simulink model "UKF"  (R2020b)
settings: Solver=VariableStepAuto  StartTime=0.0  StopTime=100  RelTol=1e-3
values from neighbouring files (symbols this model uses):
  A = [0 1 0 0; 0 0 0 0; 0 0 0 omega; 0 0 -omega 0]    [one_sine_wave.m]    (also in two_sine_wave.m = [0 1 0 0 0 0)
  acc = 0    [one_sine_wave.m]    (also in two_sine_wave.m)
  H = 100    [one_sine_wave.m]    (also in two_sine_wave.m)
libraries: sharedTrackingLibrary x3, simulink x2
settings Model: Creator=Bruger  LastModifiedBy=Bruger

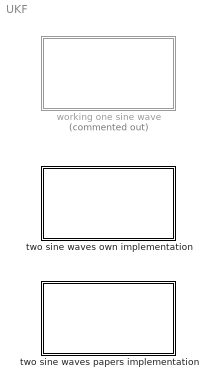
== system UKF ==
  two sine waves own implementation : Subsystem
  two sine waves papers implementation : Subsystem
  working one sine wave : Subsystem  Commented=on

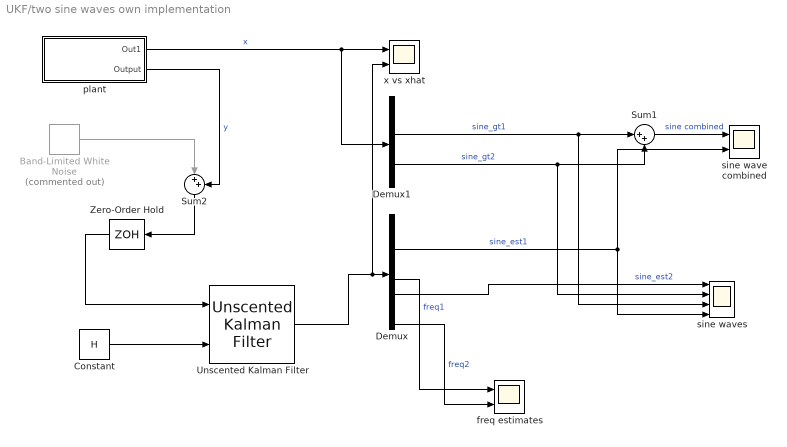
== system UKF/two sine waves own implementation ==
  Band-Limited White Noise : simulink/Sources/Band-Limited White Noise  Commented=on  Cov=[0.1]  Ts=0.05  seed=[23341]
  Constant : Constant  Value=H
  Demux : Demux  Outputs=8
  Demux1 : Demux  Outputs=6
  Sum1 : Sum  Inputs=|++
  Sum2 : Sum  Inputs=|++
  Unscented Kalman Filter : sharedTrackingLibrary/Unscented Kalman Filter  StateTransitionFcn=st_two_sine_own  HasAdditiveProcessNoise=Additive  ProcessNoise=0.1  HasTimeVaryingProcessNoise=off  HasStateTransitionFcnExtraArgument=0  InitialState=[100 0 0 20 0.5 0 40 1]  InitialStateCovariance=0.1  Alpha=1e-3  Beta=2  Kappa=0  MeasurementFcn1=meas_two_sine  HasMeasurementEnablePort1=off  HasAdditiveMeasurementNoise1=Additive  MeasurementNoise1=0.1  HasTimeVaryingMeasurementNoise1=off  HasMeasurementFcnExtraArgument1=0  MeasurementFcn2=measure_alt  HasMeasurementEnablePort2=off  HasAdditiveMeasurementNoise2=Additive  MeasurementNoise2=0.1  HasTimeVaryingMeasurementNoise2=off  HasMeasurementFcnExtraArgument2=0  MeasurementFcn3=myMeasurementFcn  HasMeasurementEnablePort3=off  HasAdditiveMeasurementNoise3=Additive  MeasurementNoise3=1  HasTimeVaryingMeasurementNoise3=off  HasMeasurementFcnExtraArgument3=0  MeasurementFcn4=myMeasurementFcn  HasMeasurementEnablePort4=off  HasAdditiveMeasurementNoise4=Additive  MeasurementNoise4=1  HasTimeVaryingMeasurementNoise4=off  HasMeasurementFcnExtraArgument4=0  MeasurementFcn5=myMeasurementFcn  HasMeasurementEnablePort5=off  HasAdditiveMeasurementNoise5=Additive  MeasurementNoise5=1  HasTimeVaryingMeasurementNoise5=off  HasMeasurementFcnExtraArgument5=0  EnableMultirate=off  StateTransitionFcnSampleTime=1  MeasurementFcn1SampleTime=1  MeasurementFcn2SampleTime=1  MeasurementFcn3SampleTime=1  MeasurementFcn4SampleTime=1  MeasurementFcn5SampleTime=1  UseCurrentEstimator=on  OutputStateCovariance=off  DataType=double  SampleTime=0.02  NumberOfMeasurements=2
      settings: SourceProductBaseCode=CT,DR,TF,ID,LP,NV,AR,RO,RR,UV,VE
  Zero-Order Hold : ZeroOrderHold  SampleTime=0.02
  freq estimates : Scope  NumInputPorts=2
  plant : Subsystem
  sine wave combined : Scope  NumInputPorts=2
  sine waves : Scope  NumInputPorts=4
  x vs xhat : Scope  NumInputPorts=2
  wires:
  Zero-Order Hold/1 -> Unscented Kalman Filter/1
  Unscented Kalman Filter/1 -> x vs xhat/2, Demux/1
  plant/1(Out1) -> x vs xhat/1, Demux1/1  "x"
  Constant/1 -> Unscented Kalman Filter/2
  Demux/6 -> sine waves/1  "sine_est2"
  Demux1/5 -> Sum1/2, sine waves/2  "sine_gt2"
  Demux/3 -> sine waves/4, sine wave combined/2  "sine_est1"
  Demux1/3 -> Sum1/1, sine waves/3  "sine_gt1"
  Demux/8 -> freq estimates/2  "freq2"
  Sum1/1 -> sine wave combined/1  "sine combined"
  Band-Limited White Noise/1 -> Sum2/1
  plant/2(Output) -> Sum2/2  "y"
  Sum2/1 -> Zero-Order Hold/1
  Demux/5 -> freq estimates/1  "freq1"

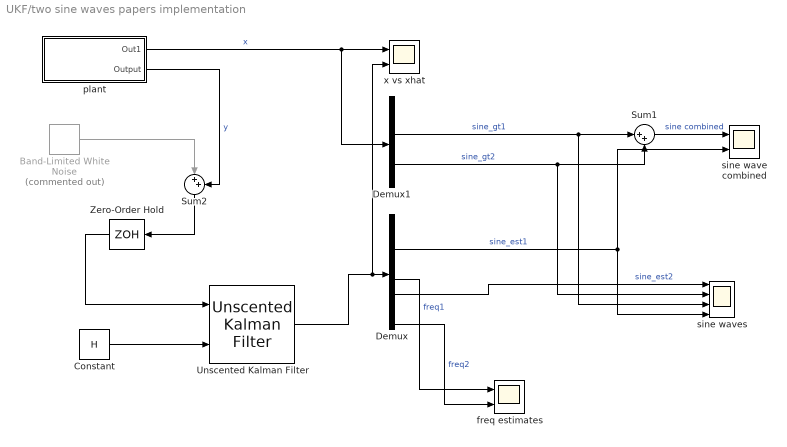
== system UKF/two sine waves papers implementation ==
  Band-Limited White Noise : simulink/Sources/Band-Limited White Noise  Commented=on  Cov=[0.1]  Ts=0.05  seed=[23341]
  Constant : Constant  Value=H
  Demux : Demux  Outputs=8
  Demux1 : Demux  Outputs=6
  Sum1 : Sum  Inputs=|++
  Sum2 : Sum  Inputs=|++
  Unscented Kalman Filter : sharedTrackingLibrary/Unscented Kalman Filter  StateTransitionFcn=st_two_sine_paper  HasAdditiveProcessNoise=Additive  ProcessNoise=0.1  HasTimeVaryingProcessNoise=off  HasStateTransitionFcnExtraArgument=0  InitialState=[100 0 0 20 0.5 0 40 1]  InitialStateCovariance=0.1  Alpha=1e-3  Beta=2  Kappa=0  MeasurementFcn1=meas_two_sine  HasMeasurementEnablePort1=off  HasAdditiveMeasurementNoise1=Additive  MeasurementNoise1=0.1  HasTimeVaryingMeasurementNoise1=off  HasMeasurementFcnExtraArgument1=0  MeasurementFcn2=measure_alt  HasMeasurementEnablePort2=off  HasAdditiveMeasurementNoise2=Additive  MeasurementNoise2=0.1  HasTimeVaryingMeasurementNoise2=off  HasMeasurementFcnExtraArgument2=0  MeasurementFcn3=myMeasurementFcn  HasMeasurementEnablePort3=off  HasAdditiveMeasurementNoise3=Additive  MeasurementNoise3=1  HasTimeVaryingMeasurementNoise3=off  HasMeasurementFcnExtraArgument3=0  MeasurementFcn4=myMeasurementFcn  HasMeasurementEnablePort4=off  HasAdditiveMeasurementNoise4=Additive  MeasurementNoise4=1  HasTimeVaryingMeasurementNoise4=off  HasMeasurementFcnExtraArgument4=0  MeasurementFcn5=myMeasurementFcn  HasMeasurementEnablePort5=off  HasAdditiveMeasurementNoise5=Additive  MeasurementNoise5=1  HasTimeVaryingMeasurementNoise5=off  HasMeasurementFcnExtraArgument5=0  EnableMultirate=off  StateTransitionFcnSampleTime=1  MeasurementFcn1SampleTime=1  MeasurementFcn2SampleTime=1  MeasurementFcn3SampleTime=1  MeasurementFcn4SampleTime=1  MeasurementFcn5SampleTime=1  UseCurrentEstimator=on  OutputStateCovariance=off  DataType=double  SampleTime=0.02  NumberOfMeasurements=2
      settings: SourceProductBaseCode=CT,DR,TF,ID,LP,NV,AR,RO,RR,UV,VE
  Zero-Order Hold : ZeroOrderHold  SampleTime=0.02
  freq estimates : Scope  NumInputPorts=2
  plant : Subsystem
  sine wave combined : Scope  NumInputPorts=2
  sine waves : Scope  NumInputPorts=4
  x vs xhat : Scope  NumInputPorts=2
  wires:
  Zero-Order Hold/1 -> Unscented Kalman Filter/1
  Unscented Kalman Filter/1 -> x vs xhat/2, Demux/1
  plant/1(Out1) -> x vs xhat/1, Demux1/1  "x"
  Constant/1 -> Unscented Kalman Filter/2
  Demux/6 -> sine waves/1  "sine_est2"
  Demux1/5 -> Sum1/2, sine waves/2  "sine_gt2"
  Demux/3 -> sine waves/4, sine wave combined/2  "sine_est1"
  Demux1/3 -> Sum1/1, sine waves/3  "sine_gt1"
  Demux/8 -> freq estimates/2  "freq2"
  Sum1/1 -> sine wave combined/1  "sine combined"
  Band-Limited White Noise/1 -> Sum2/1
  plant/2(Output) -> Sum2/2  "y"
  Sum2/1 -> Zero-Order Hold/1
  Demux/5 -> freq estimates/1  "freq1"

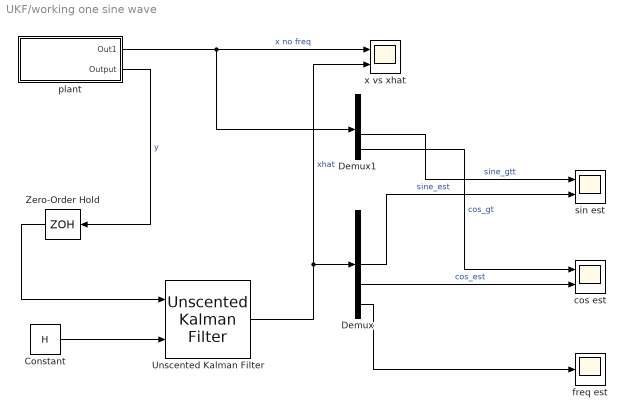
== system UKF/working one sine wave ==
  Constant : Constant  Value=H
  Demux : Demux  Outputs=5
  Demux1 : Demux
  Unscented Kalman Filter : sharedTrackingLibrary/Unscented Kalman Filter  StateTransitionFcn=st_one_sine  HasAdditiveProcessNoise=Additive  ProcessNoise=0.1  HasTimeVaryingProcessNoise=off  HasStateTransitionFcnExtraArgument=0  InitialState=[100 0 0 10 1]  InitialStateCovariance=0.1  Alpha=1e-3  Beta=2  Kappa=0  MeasurementFcn1=meas_one_sine  HasMeasurementEnablePort1=off  HasAdditiveMeasurementNoise1=Additive  MeasurementNoise1=0.1  HasTimeVaryingMeasurementNoise1=off  HasMeasurementFcnExtraArgument1=0  MeasurementFcn2=measure_alt  HasMeasurementEnablePort2=off  HasAdditiveMeasurementNoise2=Additive  MeasurementNoise2=0.1  HasTimeVaryingMeasurementNoise2=off  HasMeasurementFcnExtraArgument2=0  MeasurementFcn3=myMeasurementFcn  HasMeasurementEnablePort3=off  HasAdditiveMeasurementNoise3=Additive  MeasurementNoise3=1  HasTimeVaryingMeasurementNoise3=off  HasMeasurementFcnExtraArgument3=0  MeasurementFcn4=myMeasurementFcn  HasMeasurementEnablePort4=off  HasAdditiveMeasurementNoise4=Additive  MeasurementNoise4=1  HasTimeVaryingMeasurementNoise4=off  HasMeasurementFcnExtraArgument4=0  MeasurementFcn5=myMeasurementFcn  HasMeasurementEnablePort5=off  HasAdditiveMeasurementNoise5=Additive  MeasurementNoise5=1  HasTimeVaryingMeasurementNoise5=off  HasMeasurementFcnExtraArgument5=0  EnableMultirate=off  StateTransitionFcnSampleTime=1  MeasurementFcn1SampleTime=1  MeasurementFcn2SampleTime=1  MeasurementFcn3SampleTime=1  MeasurementFcn4SampleTime=1  MeasurementFcn5SampleTime=1  UseCurrentEstimator=on  OutputStateCovariance=off  DataType=double  SampleTime=0.1  NumberOfMeasurements=2
      settings: SourceProductBaseCode=CT,DR,TF,ID,LP,NV,AR,RO,RR,UV,VE
  Zero-Order Hold : ZeroOrderHold  SampleTime=0.1
  cos est : Scope  NumInputPorts=2
  freq est : Scope
  plant : Subsystem
  sin est : Scope  NumInputPorts=2
  x vs xhat : Scope  NumInputPorts=2
  wires:
  Zero-Order Hold/1 -> Unscented Kalman Filter/1
  plant/2(Output) -> Zero-Order Hold/1  "y"
  plant/1(Out1) -> x vs xhat/1, Demux1/1  "x no freq"
  Constant/1 -> Unscented Kalman Filter/2
  Unscented Kalman Filter/1 -> x vs xhat/2, Demux/1  "xhat"
  Demux1/4 -> cos est/1  "cos_gt"
  Demux/4 -> cos est/2  "cos_est"
  Demux1/3 -> sin est/1  "sine_gtt"
  Demux/3 -> sin est/2  "sine_est"
  Demux/5 -> freq est/1

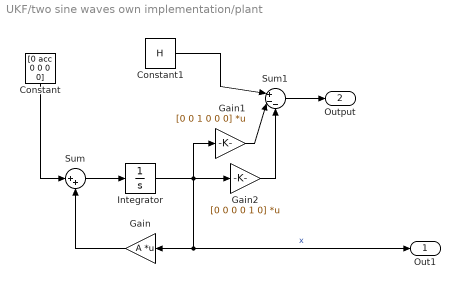
== system UKF/two sine waves own implementation/plant ==
  Constant : Constant  Value=[0 acc 0 0 0 0]
  Constant1 : Constant  Value=H
  Gain : Gain  Gain=A  Multiplication=Matrix(K*u) (u vector)
  Gain1 : Gain  Gain=[0 0 1 0 0 0]  Multiplication=Matrix(K*u) (u vector)
  Gain2 : Gain  Gain=[0 0 0 0 1 0]  Multiplication=Matrix(K*u) (u vector)
  Integrator : Integrator  InitialCondition=[H 0 0 40 0 20]
  Sum : Sum  Inputs=|++
  Sum1 : Sum  Inputs=|+--
  Out1 : Outport
  Output : Outport  Port=2
  wires:
  Integrator/1 -> Gain2/1, Gain/1, Out1/1, Gain1/1  "x"
  Gain/1 -> Sum/2
  Constant/1 -> Sum/1
  Sum/1 -> Integrator/1
  Sum1/1 -> Output/1
  Constant1/1 -> Sum1/1
  Gain1/1 -> Sum1/2
  Gain2/1 -> Sum1/3

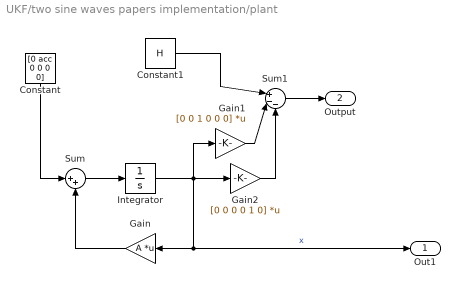
== system UKF/two sine waves papers implementation/plant ==
  Constant : Constant  Value=[0 acc 0 0 0 0]
  Constant1 : Constant  Value=H
  Gain : Gain  Gain=A  Multiplication=Matrix(K*u) (u vector)
  Gain1 : Gain  Gain=[0 0 1 0 0 0]  Multiplication=Matrix(K*u) (u vector)
  Gain2 : Gain  Gain=[0 0 0 0 1 0]  Multiplication=Matrix(K*u) (u vector)
  Integrator : Integrator  InitialCondition=[H 0 0 40 0 20]
  Sum : Sum  Inputs=|++
  Sum1 : Sum  Inputs=|+--
  Out1 : Outport
  Output : Outport  Port=2
  wires:
  Integrator/1 -> Gain2/1, Gain/1, Out1/1, Gain1/1  "x"
  Gain/1 -> Sum/2
  Constant/1 -> Sum/1
  Sum/1 -> Integrator/1
  Sum1/1 -> Output/1
  Constant1/1 -> Sum1/1
  Gain1/1 -> Sum1/2
  Gain2/1 -> Sum1/3

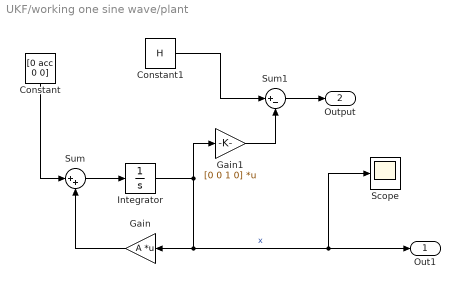
== system UKF/working one sine wave/plant ==
  Constant : Constant  Value=[0 acc 0 0]
  Constant1 : Constant  Value=H
  Gain : Gain  Gain=A  Multiplication=Matrix(K*u) (u vector)
  Gain1 : Gain  Gain=[0 0 1 0]  Multiplication=Matrix(K*u) (u vector)
  Integrator : Integrator  InitialCondition=[H 0 0 10]
  Scope : Scope
  Sum : Sum  Inputs=|++
  Sum1 : Sum  Inputs=|+-
  Out1 : Outport
  Output : Outport  Port=2
  wires:
  Integrator/1 -> Gain/1, Scope/1, Out1/1, Gain1/1  "x"
  Gain/1 -> Sum/2
  Constant/1 -> Sum/1
  Sum/1 -> Integrator/1
  Sum1/1 -> Output/1
  Constant1/1 -> Sum1/1
  Gain1/1 -> Sum1/2
